simulink model "Task1model"  (R2019a)
settings: Solver=ode15s  StartTime=0.0  StopTime=10  RelTol=1e-3
values from neighbouring files (symbols this model uses):
  delta = 15*pi/180    (= 0.261799387799)    [AuE881_HW5_Zhai_Kexuan_HW5_initialization.m]
  tireVelDesired = 20    [AuE881_HW5_Zhai_Kexuan_HW5_initialization.m]
settings Model: Creator=paredis  LastModifiedBy=kzhai

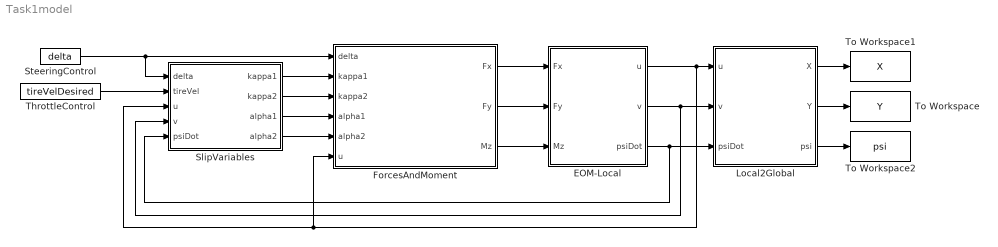
== system Task1model ==
  EOM-Local : Subsystem
  ForcesAndMoment : Subsystem
  Local2Global : Subsystem
  SlipVariables : Subsystem
  SteeringControl : Constant  Value=delta
  ThrottleControl : Constant  Value=tireVelDesired
  To Workspace : ToWorkspace  VariableName=Y  SaveFormat=Timeseries  SampleTime=-1
  To Workspace1 : ToWorkspace  VariableName=X  SaveFormat=Timeseries  SampleTime=-1
  To Workspace2 : ToWorkspace  VariableName=psi  SaveFormat=Timeseries  SampleTime=-1
  wires:
  EOM-Local/3(psiDot) -> Local2Global/3(psiDot), SlipVariables/5(psiDot)
  EOM-Local/2(v) -> Local2Global/2(v), SlipVariables/4(v)
  Local2Global/2(Y) -> To Workspace/1
  Local2Global/1(X) -> To Workspace1/1
  Local2Global/3(psi) -> To Workspace2/1
  SteeringControl/1 -> SlipVariables/1(delta), ForcesAndMoment/1(delta)
  SlipVariables/3(alpha1) -> ForcesAndMoment/4(alpha1)
  SlipVariables/4(alpha2) -> ForcesAndMoment/5(alpha2)
  ForcesAndMoment/1(Fx) -> EOM-Local/1(Fx)
  ForcesAndMoment/2(Fy) -> EOM-Local/2(Fy)
  ForcesAndMoment/3(Mz) -> EOM-Local/3(Mz)
  SlipVariables/2(kappa2) -> ForcesAndMoment/3(kappa2)
  SlipVariables/1(kappa1) -> ForcesAndMoment/2(kappa1)
  ThrottleControl/1 -> SlipVariables/2(tireVel)
  EOM-Local/1(u) -> Local2Global/1(u), ForcesAndMoment/6(u), SlipVariables/3(u)

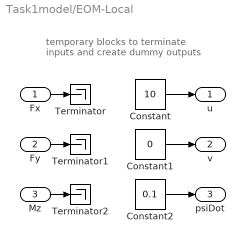
== system Task1model/EOM-Local ==
  note: temporary blocks to terminate inputs and create dummy outputs
  Fx : Inport
  Fy : Inport  Port=2
  Mz : Inport  Port=3
  Constant : Constant  Value=10
  Constant1 : Constant  Value=0
  Constant2 : Constant  Value=0.1
  Terminator : Terminator
  Terminator1 : Terminator
  Terminator2 : Terminator
  u : Outport
  v : Outport  Port=2
  psiDot : Outport  Port=3
  wires:
  Constant1/1 -> v/1
  Constant/1 -> u/1
  Fx/1 -> Terminator/1
  Mz/1 -> Terminator2/1
  Constant2/1 -> psiDot/1
  Fy/1 -> Terminator1/1

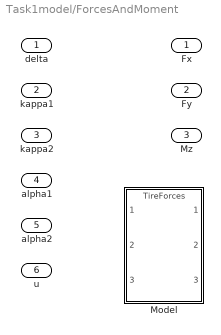
== system Task1model/ForcesAndMoment ==
  delta : Inport
  kappa1 : Inport  Port=2
  kappa2 : Inport  Port=3
  alpha1 : Inport  Port=4
  alpha2 : Inport  Port=5
  u : Inport  Port=6
  Model : ModelReference  ModelNameDialog=TireForces  SimulationMode=Normal  ModelReferenceVersion=1.12
  Fx : Outport
  Fy : Outport  Port=2
  Mz : Outport  Port=3

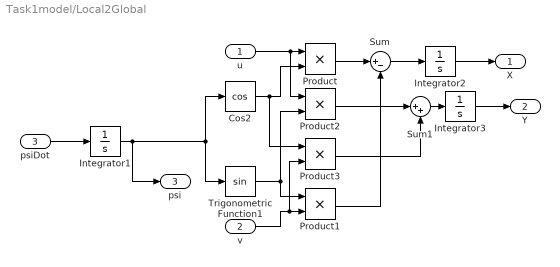
== system Task1model/Local2Global ==
  u : Inport
  v : Inport  Port=2
  psiDot : Inport  Port=3
  Cos2 : Trigonometry  Operator=cos
  Integrator1 : Integrator
  Integrator2 : Integrator
  Integrator3 : Integrator
  Product{,1..3} (4 alike) : Product
  Sum : Sum  Inputs=|+-
  Sum1 : Sum  Inputs=|++
  Trigonometric Function1 : Trigonometry
  X : Outport
  Y : Outport  Port=2
  psi : Outport  Port=3
  wires:
  psiDot/1 -> Integrator1/1
  Product1/1 -> Sum/2
  Trigonometric Function1/1 -> Product1/1, Product2/2
  Product2/1 -> Sum1/1
  Product/1 -> Sum/1
  Product3/1 -> Sum1/2
  Integrator2/1 -> X/1
  Sum/1 -> Integrator2/1
  Sum1/1 -> Integrator3/1
  v/1 -> Product3/2, Product1/2
  Cos2/1 -> Product3/1, Product/2
  Integrator3/1 -> Y/1
  u/1 -> Product2/1, Product/1
  Integrator1/1 -> Cos2/1, Trigonometric Function1/1, psi/1

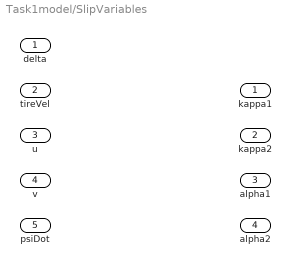
== system Task1model/SlipVariables ==
  delta : Inport
  tireVel : Inport  Port=2
  u : Inport  Port=3
  v : Inport  Port=4
  psiDot : Inport  Port=5
  kappa1 : Outport
  kappa2 : Outport  Port=2
  alpha1 : Outport  Port=3
  alpha2 : Outport  Port=4
